simulink model "Pure_Pursiut_Cntrllr"  (R2021a)
settings: Solver=FixedStepAuto  StartTime=0.0  StopTime=Ts  FixedStep=0.1  RelTol=1e-3
InitFcn:
  | Pure_Pursiut_init
values from neighbouring files (symbols this model uses):
  L = 4.7    [LCA_init.m]    (also in LCA_lateral_movie_fcn.m = 5.7; PurePursuitModelInitialization.m; Pure_Pursiut_init.m; Stanley_control_init.m)
  Ld = 10    [Pure_Pursiut_init.m]
  psi_0 = 3.9775    [PurePursuitModelInitialization.m]    (also in Pure_Pursiut_init.m = 0; Stanley_control_init.m = 0)
  Vref = 10    [Pure_Pursiut_init.m]
  X_0 = xRef(1,1)    [PurePursuitModelInitialization.m]    (also in Pure_Pursiut_init.m; Stanley_control_init.m)
  xRef = refPose(1,:)    [LCA_init.m]    (also in MPC_init.m; PurePursuitModelInitialization.m = refPose(:,1); Pure_Pursiut_init.m; Stanley_control_init.m = refpose(1,:))
  Y_0 = yRef(1,2)    [PurePursuitModelInitialization.m]    (also in Pure_Pursiut_init.m = yRef(1,1); Stanley_control_init.m = yRef(1,1))
  yRef = refPose(2,:) + 2    [LCA_init.m]    (also in MPC_init.m; PurePursuitModelInitialization.m = -refPose(:,2); Pure_Pursiut_init.m = refPose(2,:); Stanley_control_init.m = refpose(2,:))
libraries: robotalgslib x1, autolibshared x1
settings Model: Creator=User  LastModifiedBy=User

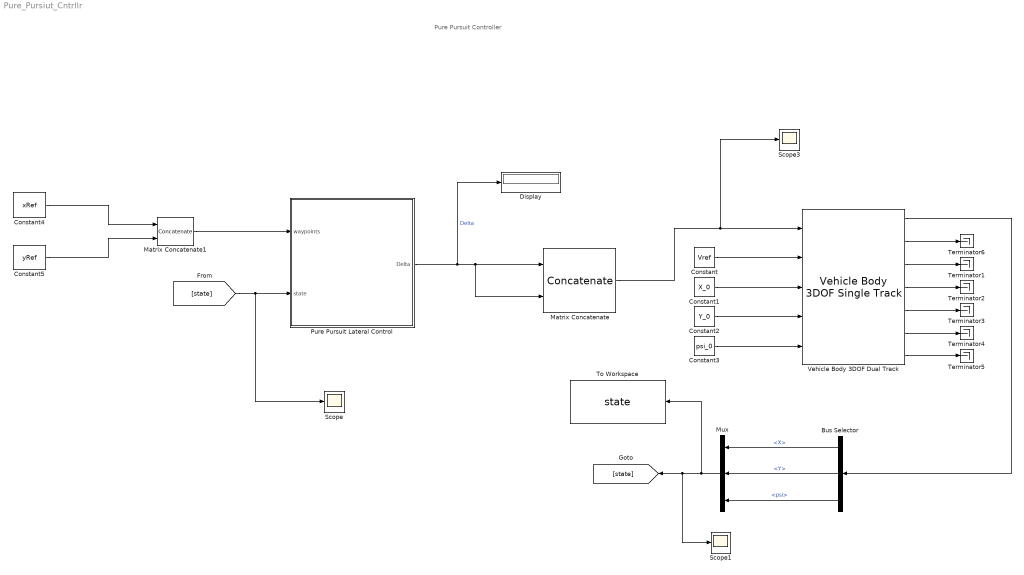
== system Pure_Pursiut_Cntrllr ==
  note: Pure Pursuit Controller
  Bus Selector : BusSelector  OutputSignals=InertFrm.Cg.Disp.X,InertFrm.Cg.Disp.Y,InertFrm.Cg.Ang.psi
  Constant : Constant  Value=Vref
  Constant1 : Constant  Value=X_0
  Constant2 : Constant  Value=Y_0
  Constant3 : Constant  Value=psi_0
  Constant4 : Constant  Value=xRef  SampleTime=0.1
  Constant5 : Constant  Value=yRef  SampleTime=0.1
  Display : Display
  Matrix Concatenate : Concatenate  ConcatenateDimension=2
  Matrix Concatenate1 : Concatenate  Mode=Multidimensional array  ConcatenateDimension=2
  Mux : Mux  Inputs=3
  Pure Pursuit Lateral Control : Subsystem
  Scope : Scope
  Scope1 : Scope
  Scope3 : Scope
  Terminator{1..6} (6 alike) : Terminator
  To Workspace : ToWorkspace  VariableName=state  SampleTime=-1
      settings: Save2DSignal=2-D array (concatenate along first dimension)
  Vehicle Body 3DOF Dual Track : autolibshared/Vehicle Body 3DOF Single Track  trackMode=Dual  inputMode=External longitudinal velocity  frontSteerMode=on  rearSteerMode=off  windMode=off  muMode=off  extFMode=off  extMMode=off  htchFMode=off  htchMMode=off  extXo=on  extpsio=on  extxdoto=off  extro=off  extYo=on  extTamb=off  extydoto=off  aMode=2  NF=2  NR=2  m=2000  a=1.4  b=1.6  h=0.35  dh=1  hh=0.2  X_o=0  xdot_o=0  CalphaMode=off  sigmaMode=on  d=0  hl=0  w=[1.4,1.4]  Cy_f=12e3  Cy_r=11e3  sigma_f=.1  sigma_r=.1  alpha_f_brk=[-.1 .1]  Cy_f_data=[-9e3 9e3]  alpha_r_brk=[-.1 .1]  Cy_r_data=[-9e3 9e3]  Y_o=0  ydot_o=0  Izz=4000  psi_o=0  r_o=0  Af=2  Cd=.3  Cl=.1  Cpm=.1  beta_w=[0:0.01:0.3]  Cs=[0:0.03:0.9]  Cym=[0:0.01:0.3]  Pabs=101325  Tair=273  g=9.81  mu=1  xdot_tol=.01  Fznom=5000  Fxtire_sat=7e4  Fytire_sat=7e4  longOff=0  latOff=0  vertOff=0  wrapAng=off
      settings: SourceProductBaseCode=PW,DR,MT,UV,VE
  wires:
  Pure Pursuit Lateral Control/1(Delta) -> Display/1, Matrix Concatenate/2, Matrix Concatenate/1  "Delta"
  Matrix Concatenate/1 -> Scope3/1, Vehicle Body 3DOF Dual Track/1
  Constant/1 -> Vehicle Body 3DOF Dual Track/2
  Constant1/1 -> Vehicle Body 3DOF Dual Track/3
  Constant2/1 -> Vehicle Body 3DOF Dual Track/4
  Constant3/1 -> Vehicle Body 3DOF Dual Track/5
  Vehicle Body 3DOF Dual Track/2 -> Terminator6/1
  Vehicle Body 3DOF Dual Track/3 -> Terminator1/1
  Vehicle Body 3DOF Dual Track/4 -> Terminator2/1
  Vehicle Body 3DOF Dual Track/5 -> Terminator3/1
  Vehicle Body 3DOF Dual Track/6 -> Terminator4/1
  Vehicle Body 3DOF Dual Track/7 -> Terminator5/1
  Mux/1 -> To Workspace/1, Scope1/1, [state]
  [state] -> Scope/1, Pure Pursuit Lateral Control/2(state)
  Constant5/1 -> Matrix Concatenate1/2
  Constant4/1 -> Matrix Concatenate1/1
  Vehicle Body 3DOF Dual Track/1 -> Bus Selector/1
  Bus Selector/1 -> Mux/1  "<X>"
  Bus Selector/2 -> Mux/2  "<Y>"
  Bus Selector/3 -> Mux/3  "<psi>"
  Matrix Concatenate1/1 -> Pure Pursuit Lateral Control/1(waypoints)

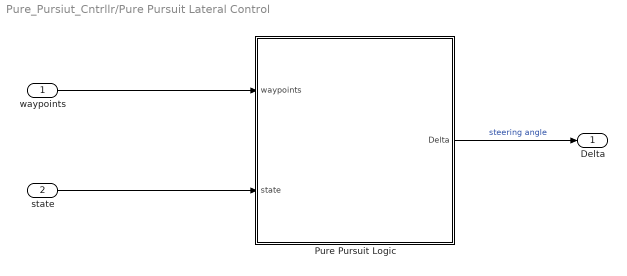
== system Pure_Pursiut_Cntrllr/Pure Pursuit Lateral Control ==
  waypoints : Inport
  state : Inport  Port=2
  Pure Pursuit Logic : Subsystem
  Delta : Outport
  wires:
  Pure Pursuit Logic/1(Delta) -> Delta/1  "steering angle"
  waypoints/1 -> Pure Pursuit Logic/1(waypoints)
  state/1 -> Pure Pursuit Logic/2(state)

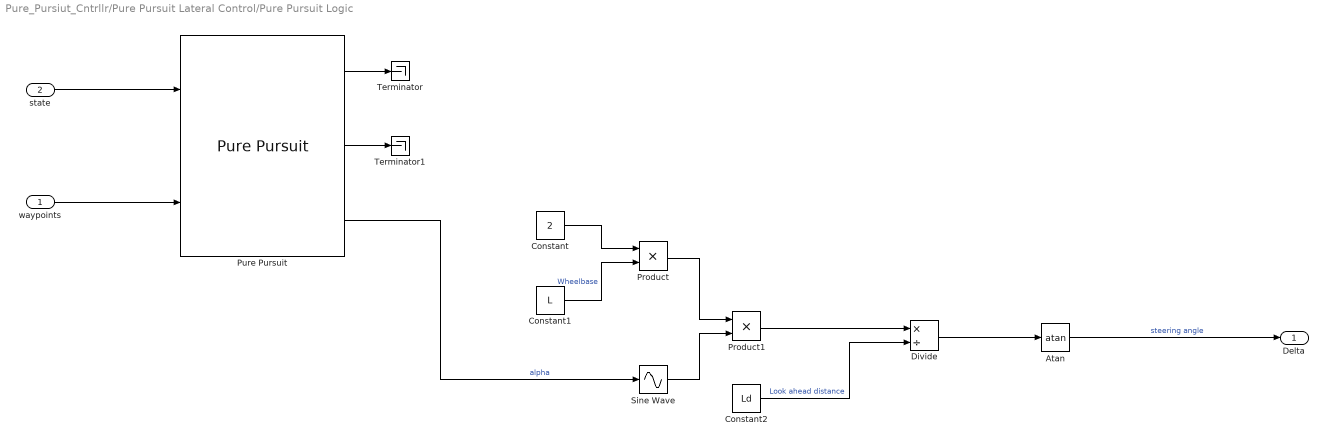
== system Pure_Pursiut_Cntrllr/Pure Pursuit Lateral Control/Pure Pursuit Logic ==
  waypoints : Inport
  state : Inport  Port=2
  Atan : Trigonometry  Operator=atan
  Constant : Constant  Value=2
  Constant1 : Constant  Value=L
  Constant2 : Constant  Value=Ld
  Divide : Product  Inputs=*/
  Product : Product
  Product1 : Product
  Pure Pursuit : robotalgslib/Pure Pursuit  DesiredLinearVelocity=Vref  MaxAngularVelocity=1.0  LookaheadDistance=Ld  TargetDirPort=on  SimulateUsing=Code generation
  Sine Wave : Sin  TimeSource=Use external signal  SampleTime=0
  Terminator : Terminator
  Terminator1 : Terminator
  Delta : Outport
  wires:
  state/1 -> Pure Pursuit/1
  waypoints/1 -> Pure Pursuit/2
  Pure Pursuit/1 -> Terminator/1
  Pure Pursuit/2 -> Terminator1/1
  Pure Pursuit/3 -> Sine Wave/1  "alpha"
  Constant/1 -> Product/1
  Constant1/1 -> Product/2  "Wheelbase"
  Product/1 -> Product1/1
  Sine Wave/1 -> Product1/2
  Product1/1 -> Divide/1
  Constant2/1 -> Divide/2  "Look ahead distance"
  Divide/1 -> Atan/1
  Atan/1 -> Delta/1  "steering angle"
